simulink model "exampleHelperAvoidObstaclesMobileRobot"  (R2024a)
settings: Solver=VariableStepAuto  StartTime=0.0  StopTime=1000  RelTol=1e-3
undefined symbols (not defined in the file): initTheta, initX, initY, lidarNoiseSeeds, lidarNoiseVariance, mapMatrix, maxAngSpeed, maxLinSpeed, maxRange, sampleTime
libraries: simulink x3, mcbcontrolslib x2, rllib x1, robotmobilelib x1
settings Model: Creator=The MathWorks, Inc.  LastModifiedBy=kevin
settings SolverCC: AlgebraicLoopSolver=TrustRegion
settings DebuggingCC: ParameterOverflowMsg=warning  ParameterUnderflowMsg=warning  UnconnectedInputMsg=warning  UnconnectedOutputMsg=warning  UnconnectedLineMsg=warning
settings ModelReferenceCC: EnableRefExpFcnMdlSchedulingChecks=on
settings RTWCC: GPUComputeCapability=3.5
settings ConfigComp: DVTestSuiteOptimization=Auto  DVDetectOutOfBounds=on  DVModelReferenceHarness=on  DVHarnessSource=Signal Editor

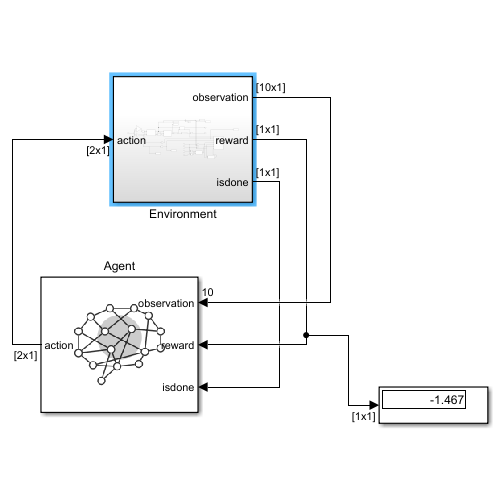
[thumbnail: Simulink's stored preview of the top-level diagram]
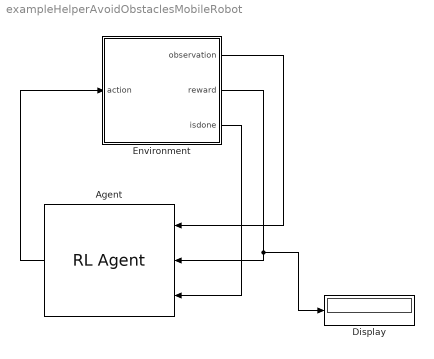
== system exampleHelperAvoidObstaclesMobileRobot ==
  Agent : rllib/RL Agent  Agent=obstacleAvoidanceAgent  ExternalActionAsInput=off  ProvideLastAction=off  ProvideCumRwd=off  TreatAsDirectFeedthrough=on  UseStrictObservationDataTypes=off
  Display : Display
  Environment : Subsystem
  wires:
  Environment/1(observation) -> Agent/1
  Environment/2(reward) -> Agent/2, Display/1
  Environment/3(isdone) -> Agent/3
  Agent/1 -> Environment/1(action)

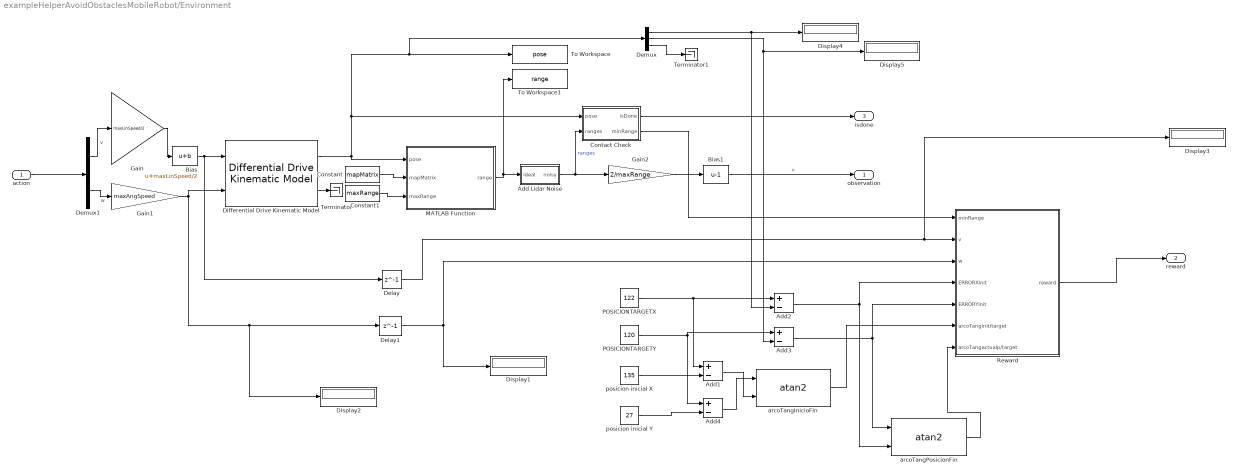
== system exampleHelperAvoidObstaclesMobileRobot/Environment ==
  action : Inport
  Add Lidar Noise : Subsystem
  Add{1..4} (4 alike) : Sum  Inputs=+-
  Bias : Bias  Bias=maxLinSpeed/2  SaturateOnIntegerOverflow=off
  Bias1 : Bias  Bias=-1  SaturateOnIntegerOverflow=off
  Constant : Constant  Value=mapMatrix
  Constant1 : Constant  Value=maxRange
  Contact Check : Subsystem
  Delay : Delay  DelayLength=1  InitialCondition=0  UseCircularBuffer=on
  Delay1 : Delay  DelayLength=1  InitialCondition=0  UseCircularBuffer=on
  Demux : Demux  Outputs=3
  Demux1 : Demux  Outputs=2
  Differential Drive Kinematic Model : robotmobilelib/Differential Drive Kinematic Model  VehicleInputs=Vehicle Speed & Heading Angular Velocity  WheelRadius=0.05  WheelSpeedRange=[-inf inf]  TrackWidth=0.2  InitialState=[initX; initY; initTheta]  SimulateUsing=Code generation
  Display{1..5} (5 alike) : Display
  Gain : Gain  Gain=maxLinSpeed/2
  Gain1 : Gain  Gain=maxAngSpeed
  Gain2 : Gain  Gain=2/maxRange
  MATLAB Function : MATLAB Function  TreatAsAtomicUnit=on
  POSICIONTARGETX : Constant  Value=122
  POSICIONTARGETY : Constant  Value=120
  Reward : Subsystem
  Terminator : Terminator
  Terminator1 : Terminator
  To Workspace : ToWorkspace  VariableName=pose  SampleTime=-1
      settings: Save2DSignal=2-D array (concatenate along first dimension)
  To Workspace1 : ToWorkspace  VariableName=range  SampleTime=-1
  arcoTangInicioFin : mcbcontrolslib/atan2  ApproximationMethod=None  NumberOfIterations=11  NumberOfDataPoints=16  InterpMethod=Flat  outputUnit=Radians  TableDataTypeStr=Inherit: Inherit via input
      settings: LibrarySourceBlock=mcblib/Controls/Math Transforms/atan2
  arcoTangPosicionFin : mcbcontrolslib/atan2  ApproximationMethod=None  NumberOfIterations=11  NumberOfDataPoints=16  InterpMethod=Flat  outputUnit=Radians  TableDataTypeStr=Inherit: Inherit via input
      settings: LibrarySourceBlock=mcblib/Controls/Math Transforms/atan2
  posicion inicial X : Constant  Value=135
  posicion inicial Y : Constant  Value=27
  observation : Outport
  reward : Outport  Port=2
  isdone : Outport  Port=3
  wires:
  Differential Drive Kinematic Model/2 -> Terminator/1
  Constant/1 -> MATLAB Function/2(mapMatrix)
  Differential Drive Kinematic Model/1 -> Demux/1, To Workspace/1, Contact Check/1(pose), MATLAB Function/1(pose)
  action/1 -> Demux1/1
  Bias/1 -> Delay/1, Differential Drive Kinematic Model/1
  Gain1/1 -> Differential Drive Kinematic Model/2, Display2/1, Delay1/1
  MATLAB Function/1(range) -> To Workspace1/1, Add Lidar Noise/1(ideal)
  Contact Check/1(isDone) -> isdone/1
  Contact Check/2(minRange) -> Reward/1(minRange)
  Reward/1(reward) -> reward/1
  Gain2/1 -> Bias1/1
  Bias1/1 -> observation/1  "v"
  Constant1/1 -> MATLAB Function/3(maxRange)
  Delay/1 -> Display3/1, Reward/2(v)
  Delay1/1 -> Display1/1, Reward/3(w)
  Demux1/2 -> Gain1/1  "w"
  Gain/1 -> Bias/1
  Demux1/1 -> Gain/1  "v"
  Add Lidar Noise/1(noisy) -> Gain2/1, Contact Check/2(ranges)  "ranges"
  POSICIONTARGETX/1 -> Add1/1, Add2/1
  POSICIONTARGETY/1 -> Add3/1, Add4/1
  Demux/3 -> Terminator1/1
  Demux/1 -> Display4/1, Add2/2
  Demux/2 -> Add3/2, Display5/1
  Add2/1 -> arcoTangPosicionFin/2, Reward/4(ERRORXinit)
  Add3/1 -> arcoTangPosicionFin/1, Reward/5(ERRORYinit)
  posicion inicial X/1 -> Add1/2
  posicion inicial Y/1 -> Add4/2
  Add4/1 -> arcoTangInicioFin/1
  Add1/1 -> arcoTangInicioFin/2
  arcoTangInicioFin/1 -> Reward/6(arcoTanginit/target)
  arcoTangPosicionFin/1 -> Reward/7(arcoTangactualp/target)

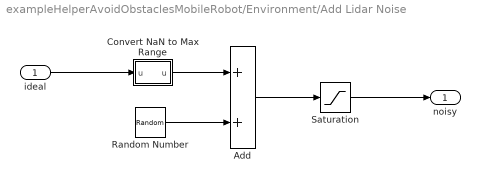
== system exampleHelperAvoidObstaclesMobileRobot/Environment/Add Lidar Noise ==
  ideal : Inport
  Add : Sum
  Convert NaN to Max Range : MATLAB Function  TreatAsAtomicUnit=on
  Random Number : RandomNumber  Variance=lidarNoiseVariance  Seed=lidarNoiseSeeds  SampleTime=sampleTime
  Saturation : Saturate  UpperLimit=inf  LowerLimit=0
  noisy : Outport
  wires:
  Random Number/1 -> Add/2
  Add/1 -> Saturation/1
  Saturation/1 -> noisy/1
  ideal/1 -> Convert NaN to Max Range/1("u ")
  Convert NaN to Max Range/1(u) -> Add/1

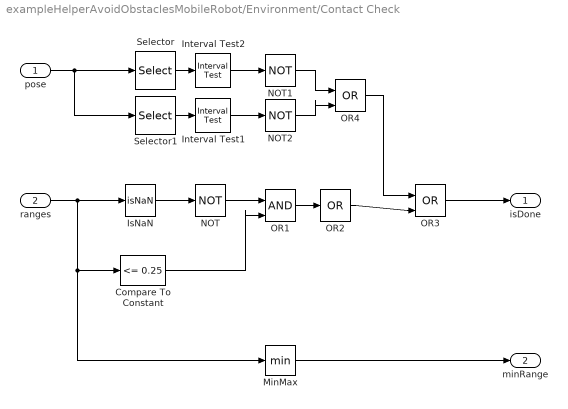
== system exampleHelperAvoidObstaclesMobileRobot/Environment/Contact Check ==
  pose : Inport
  ranges : Inport  Port=2
  Compare To Constant : simulink/Logic and Bit Operations/Compare To Constant  relop=<=  const=0.25  OutDataTypeStr=boolean
  Interval Test1 : simulink/Logic and Bit Operations/Interval Test  IntervalClosedRight=on  uplimit=size(mapMatrix, 1)  IntervalClosedLeft=on  lowlimit=0  OutDataTypeStr=boolean
  Interval Test2 : simulink/Logic and Bit Operations/Interval Test  IntervalClosedRight=on  uplimit=size(mapMatrix, 2)  IntervalClosedLeft=on  lowlimit=0  OutDataTypeStr=boolean
  IsNaN : RelationalOperator  Operator=isNaN  OutDataTypeStr=boolean  RndMeth=Simplest  InputSameDT=off
  MinMax : MinMax
  NOT : Logic  Operator=NOT  IconShape=distinctive  AllPortsSameDT=off  OutDataTypeStr=boolean
  NOT1 : Logic  Operator=NOT  IconShape=distinctive  AllPortsSameDT=off  OutDataTypeStr=boolean
  NOT2 : Logic  Operator=NOT  IconShape=distinctive  AllPortsSameDT=off  OutDataTypeStr=boolean
  OR1 : Logic  IconShape=distinctive  AllPortsSameDT=off  OutDataTypeStr=boolean
  OR2 : Logic  Operator=OR  Inputs=1  IconShape=distinctive  AllPortsSameDT=off  OutDataTypeStr=boolean
  OR3 : Logic  Operator=OR  IconShape=distinctive  AllPortsSameDT=off  OutDataTypeStr=boolean
  OR4 : Logic  Operator=OR  IconShape=distinctive  AllPortsSameDT=off  OutDataTypeStr=boolean
  Selector : Selector  InputPortWidth=3  IndexOptions=Index vector (dialog)  Indices=1  OutputSizes=1
  Selector1 : Selector  InputPortWidth=3  IndexOptions=Index vector (dialog)  Indices=2  OutputSizes=1
  isDone : Outport  VectorParamsAs1DForOutWhenUnconnected=off
  minRange : Outport  Port=2  VectorParamsAs1DForOutWhenUnconnected=off
  wires:
  OR1/1 -> OR2/1
  Compare To Constant/1 -> OR1/2
  NOT/1 -> OR1/1
  ranges/1 -> MinMax/1, Compare To Constant/1, IsNaN/1
  IsNaN/1 -> NOT/1
  MinMax/1 -> minRange/1
  OR3/1 -> isDone/1
  pose/1 -> Selector/1, Selector1/1
  Selector/1 -> Interval Test2/1
  Selector1/1 -> Interval Test1/1
  OR2/1 -> OR3/2
  NOT1/1 -> OR4/1
  Interval Test1/1 -> NOT2/1
  OR4/1 -> OR3/1
  Interval Test2/1 -> NOT1/1
  NOT2/1 -> OR4/2

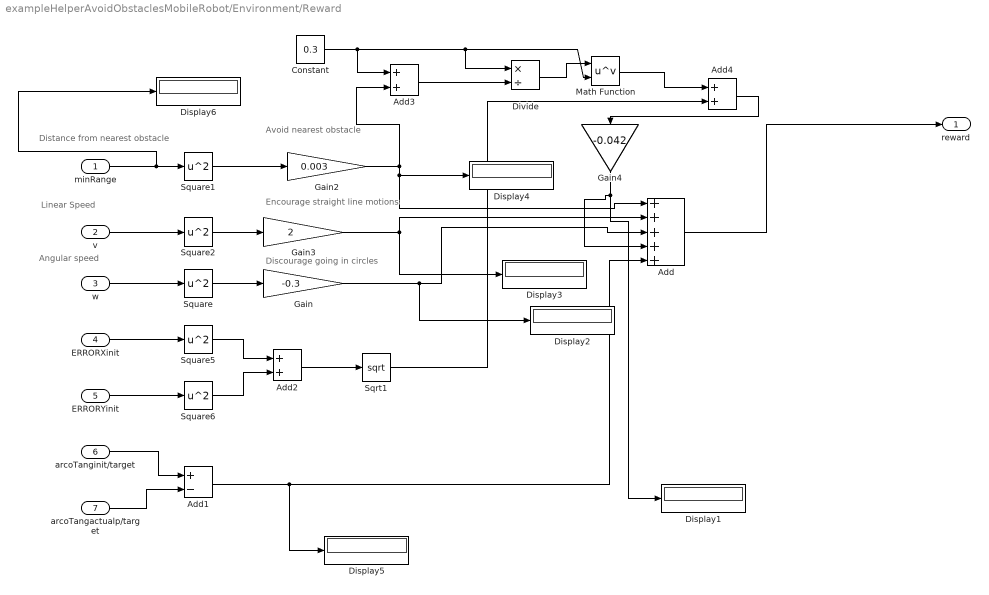
== system exampleHelperAvoidObstaclesMobileRobot/Environment/Reward ==
  note: Discourage going in circles
  note: Encourage straight line motions
  note: Angular speed
  note: Linear Speed
  note: Distance from nearest obstacle
  note: Avoid nearest obstacle
  minRange : Inport
  v : Inport  Port=2
  w : Inport  Port=3
  ERRORXinit : Inport  Port=4
  ERRORYinit : Inport  Port=5
  arcoTanginit/target : Inport  Port=6
  arcoTangactualp/target : Inport  Port=7
  Add : Sum  Inputs=+++++
  Add1 : Sum  Inputs=+-
  Add2 : Sum
  Add3 : Sum
  Add4 : Sum
  Constant : Constant  Value=0.3
  Display{1..6} (6 alike) : Display
  Divide : Product  Inputs=*/
  Gain : Gain  Gain=-0.3
  Gain2 : Gain  Gain=0.003
  Gain3 : Gain  Gain=2
  Gain4 : Gain  Gain=-0.042
  Math Function : Math  Operator=pow
  Sqrt1 : Sqrt
  Square{,1..2,5..6} (5 alike) : Math  Operator=square  SignedPower=on
  reward : Outport  VectorParamsAs1DForOutWhenUnconnected=off
  wires:
  Square/1 -> Gain/1
  w/1 -> Square/1
  Gain/1 -> Display2/1, Add/3
  minRange/1 -> Display6/1, Square1/1
  Gain2/1 -> Display4/1, Add/1, Add3/2
  Square1/1 -> Gain2/1
  v/1 -> Square2/1
  Square2/1 -> Gain3/1
  Gain3/1 -> Display3/1, Add/2
  Add/1 -> reward/1
  ERRORXinit/1 -> Square5/1
  ERRORYinit/1 -> Square6/1
  Square5/1 -> Add2/1
  Square6/1 -> Add2/2
  Add2/1 -> Sqrt1/1
  arcoTanginit/target/1 -> Add1/1
  arcoTangactualp/target/1 -> Add1/2
  Add1/1 -> Display5/1, Add/5
  Constant/1 -> Add3/1, Math Function/2, Divide/1
  Add3/1 -> Divide/2
  Divide/1 -> Math Function/1
  Math Function/1 -> Add4/1
  Sqrt1/1 -> Add4/2
  Add4/1 -> Gain4/1
  Gain4/1 -> Display1/1, Add/4

== matlab function exampleHelperAvoidObstaclesMobileRobot/Environment/MATLAB Function ==
  settings: updateMethod=DISCRETE
  data: range output size=[10, 1]; pose input size=[3, 1]; mapMatrix input size=[size(mapMatrix, 1), size(mapMatrix, 2)]; maxRange input; mapScale parameter
function range = RangeSensor(pose, mapMatrix, maxRange, mapScale)
range=exampleHelperAvoidObstaclesRangeSensor(pose,mapMatrix,maxRange,mapScale);

== matlab function exampleHelperAvoidObstaclesMobileRobot/Environment/Add Lidar Noise/Convert NaN to Max Range ==
  data: u input; u output; maxRange parameter
function u = removeNans(u,maxRange)

u(isnan(u)) = maxRange;
